simulink model "controllerLogicSim"  (R2017a)
settings: Solver=ode23t  StartTime=0.0  StopTime=27.5  FixedStep=0.001  MaxStep=0.0001  RelTol=1e-3
undefined symbols (not defined in the file): sigbuilder_block
settings Model: Creator=usuario  LastModifiedBy=Carlos María
settings DebuggingCC: SFNoUnconditionalDefaultTransitionDiag=warning

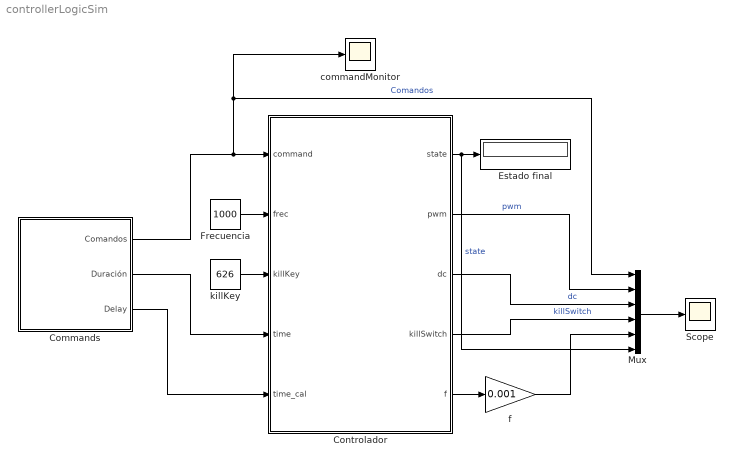
== system controllerLogicSim ==
  Commands : Subsystem  Tag=STV Subsys  LoadFcn=sigbuilder_block('load');  StartFcn=sigbuilder_block('start');  StopFcn=sigbuilder_block('stop');  ClipboardFcn=sigbuilder_block('clipboard');  mask(Sigbuilder block){tuvar=[0:10]}
      mask help: Simulink:masks:SigbuilderBlock_MD
      mask init:
      | if ~strcmp(get_param(bdroot(gcbh),'SimulationStatus'),'stopped') tuvar = sigbuilder_block('maskInit'); end
      settings: CopyFcn=sigbuilder_block('copy');  DeleteFcn=sigbuilder_block('delete');  ModelCloseFcn=sigbuilder_block('modelClose');  PreSaveFcn=sigbuilder_block('preSave');  PauseFcn=sigbuilder_block('pause');  ContinueFcn=sigbuilder_block('continue');  NameChangeFcn=sigbuilder_block('namechange');  OpenFcn=sigbuilder_block('open',[87 94.8 642.6 428.4 ]);  CloseFcn=sigbuilder_block('close');
      mask Display: plot(0, 0, 100, 100,[2, 2, 32, 32, 2], [68, 8, 8, 68, 68],[32, 2], [38, 38], [32, 19, 2],[53, 60, 44], [32, 17, 17, 2],[16, 16, 31, 31]);txt = getActiveGroup(gcbh);text(2, 100, txt,'verticalAlignment', 'top');
  Controlador : Stateflow chart  TreatAsAtomicUnit=on
  Estado final : Display
  Frecuencia : Constant  Value=1000
  Mux : Mux  Inputs=6
  Scope : Scope
  commandMonitor : Scope
  f : Gain  Gain=0.001
  killKey : Constant  Value=626
  wires:
  Frecuencia/1 -> Controlador/2(frec)
  Mux/1 -> Scope/1
  killKey/1 -> Controlador/3(killKey)
  Commands/1(Comandos) -> Controlador/1(command), Mux/1, commandMonitor/1  "Comandos"
  Controlador/1(state) -> Mux/6, Estado final/1  "state"
  Controlador/2(pwm) -> Mux/2  "pwm"
  Controlador/3(dc) -> Mux/3  "dc"
  Controlador/4(killSwitch) -> Mux/4  "killSwitch"
  Controlador/5(f) -> f/1
  f/1 -> Mux/5
  Commands/2(Duración) -> Controlador/4(time)
  Commands/3(Delay) -> Controlador/5(time_cal)

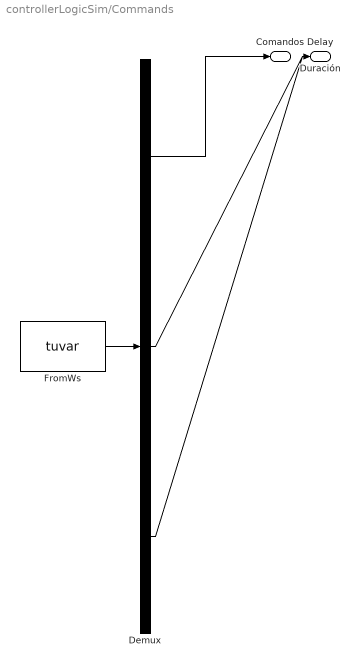
== system controllerLogicSim/Commands ==
  Demux : Demux  Tag=STV Demux  Outputs=3
  FromWs : FromWorkspace  Tag=STV FromWs  VariableName=tuvar  SampleTime=0
      SigBuilderData=|
      | common.afterFinalStr = 'Extrapolate'
      | common.sampleTime = 0
      | dataSet.timeRange = [0 25]
      | dataSet.name = 'Group 1'
      | sbobj.Groups.Name = 'Group 1'
      | sbobj.Groups.Signals(1).Name = 'Comandos'
      | sbobj.Groups.Signals(1).XData = [0 1 1 2 2 3 3 4 4 5 5 8 8 9 9 10 10 13 13 14 14 23 23 23.5 23.5 25]
      | sbobj.Groups.Signals(1).YData = [0 0 2 2 1 1 0 0 3 3 0 0 1 1 4 4 0 0 5 5 0 0 6 6 0 0]
      | sbobj.Groups.Signals(2).Name = 'Duración'
      | sbobj.Groups.Signals(2).XData = [0 9 9 10 10 13 13 14 14 25]
      | sbobj.Groups.Signals(2).YData = [0 0 3 3 0 0 4 4 0 0]
      | sbobj.Groups.Signals(3).Name = 'Delay'
      | sbobj.Groups.Signals(3).XData = [0 4 4 5 5 13 13 14 14 25]
      | sbobj.Groups.Signals(3).YData = [0 0 2 2 0 0 3 3 0 0]
      | sbobj.Groups.TimeRange = [0 25]
  Comandos : Outport  Tag=STV Outport
  Duración : Outport  Tag=STV Outport  Port=2
  Delay : Outport  Tag=STV Outport  Port=3
  wires:
  Demux/1 -> Comandos/1
  FromWs/1 -> Demux/1
  Demux/2 -> Duración/1
  Demux/3 -> Delay/1

== stateflow chart controllerLogicSim/Controlador ==
  state On
    state OnTimed
      entry:
      f=frec;
      dc=0.75;
      pwm=1;
      state=aux;
      d=time;
      on after(d,sec):
      offFlag=1;
    state On
      entry:
      f=frec;
      dc=0.75;
      pwm=1;
      state=aux;
    (default) -> (junction 28)
    (junction 28) -> On.On [order 1] : [aux==2]
    (junction 28) -> OnTimed [order 2] : [aux==4]
  note: off				1
      | on				2
      | onCal			3
      | timedOn		4
      | timedOnCal 	5
      | kill 				6
      | setKey 		7
      | telemetry 		8
      | VATinit/null 	0
  state Scheduled
    state auxTimedCal
    state OnTimedCal
      entry:
      state=aux;
      f=frec;
      dc=0.75;
      pwm=1;
      offFlag=0;
      on after(d,sec):
      offFlag=1;
    state OnCal
      entry:
      state=aux;
      on after(cal,sec):
      f=frec;
      dc=0.75;
      pwm=1;
      state=aux;
    (default) -> (junction 54) : {cal=time_cal}
    (junction 54) -> auxTimedCal [order 2] : [aux == 5]{state=5; d=time}
    (junction 54) -> OnCal [order 1] : [aux==3]
    auxTimedCal -> OnTimedCal : after(cal,sec)
  state VATinit
    entry:
    key=626;
    p=0;
    state=0;
    aux=0;
    killSwitch=0;
    during:
    p=1;
  state Off
    entry:
    f=0;
    dc=0;
    pwm=0;
    state=1;
    offFlag=0;
    aux=0;
    cal=0;
    d=0;
  state Dead
    entry:
    killSwitch = 1;
    p=0;
    f=0;
    dc=0;
    pwm=0;
    state=6;
    offFlag=0;
    cal=0;
    d=0;
  On -> Dead [order 2] : [command == 6 && killKey == key]
  Off -> On [order 1] : [command == 2 || command == 4]{aux=command}
  On -> Off [order 1] : [offFlag == 1 || command == 1]
  Off -> Scheduled [order 2] : [command == 3||command == 5]{aux = command}
  (default) -> VATinit
  VATinit -> Off : [p~=0]
  Scheduled -> Off [order 1] : [command == 1 || offFlag == 1]
  Off -> Dead [order 3] : [command == 6 && killKey == key]
  Scheduled -> Dead [order 2] : [command == 6 && killKey == key]
  Dead -> Dead : [command ~=0]{p=1}
  data: command input; frec input; state output; pwm output; dc output; offFlag local; p local; aux local; key local; killKey input; killSwitch output; f output; time input; d local; time_cal input; cal local
